simulink model "imc_simu"  (R2023b)
settings: Solver=VariableStepAuto  StartTime=0.0  StopTime=10.0  RelTol=1e-3
settings Model: Creator=Administrator  LastModifiedBy=Administrator

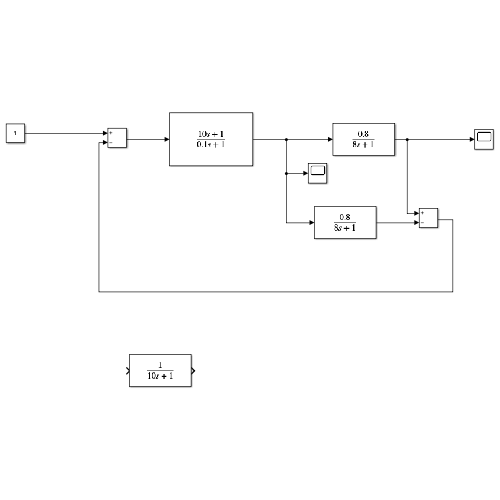
[thumbnail: Simulink's stored preview of the top-level diagram]
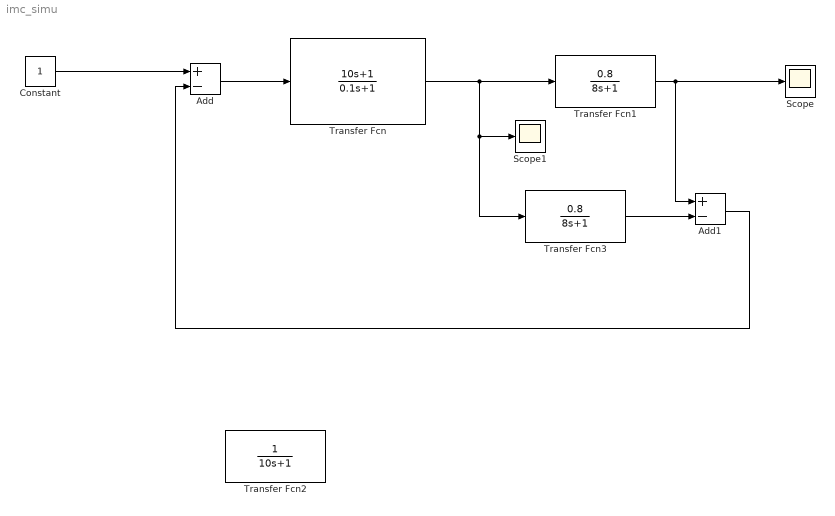
== system imc_simu ==
  Add : Sum  Inputs=+-
  Add1 : Sum  Inputs=+-
  Constant : Constant
  Scope : Scope
  Scope1 : Scope
  Transfer Fcn : TransferFcn  Numerator=[10 1]  Denominator=[0.1 1]
  Transfer Fcn1 : TransferFcn  Numerator=[0.8]  Denominator=[8 1]
  Transfer Fcn2 : TransferFcn  Denominator=[10 1]
  Transfer Fcn3 : TransferFcn  Numerator=[0.8]  Denominator=[8 1]
  wires:
  Add/1 -> Transfer Fcn/1
  Transfer Fcn/1 -> Transfer Fcn3/1, Scope1/1, Transfer Fcn1/1
  Transfer Fcn3/1 -> Add1/2
  Transfer Fcn1/1 -> Scope/1, Add1/1
  Add1/1 -> Add/2
  Constant/1 -> Add/1
